simulink model "Assignment_lego"  (R2023b)
settings: Solver=FixedStepAuto  StartTime=0.0  StopTime=10  RelTol=1e-3  EnableMultiTasking=on
libraries: legoev3lib x7
settings Model: ExtModeBatchMode=on  ExtModeTrigDuration=2  Creator=Krish  LastModifiedBy=Krish
settings SolverCC: PositivePriorityOrder=on  AutoInsertRateTranBlk=on
settings OptimizationCC: EnhancedBackFolding=on  PassReuseOutputArgsAs=Individual arguments  ZeroExternalMemoryAtStartup=off  ZeroInternalMemoryAtStartup=off  MaxStackSize=64  OptimizeBlockOrder=speed  DifferentSizesBufferReuse=on  OptimizationCustomize=off  EfficientTunableParamExpr=on
settings DebuggingCC: ParameterTunabilityLossMsg=error
settings HardwareCC: ProdBitPerPointer=32  ProdBitPerSizeT=32  ProdBitPerPtrDiffT=32  ProdLargestAtomicInteger=Long  ProdWordSize=32  ProdHWDeviceType=ARM Compatible->ARM 9
settings SFSimCC: MATLABDynamicMemAlloc=off
settings RTWCC: Description=Embedded Coder  SystemTargetFile=ert.tlc  HardwareBoard=LEGO MINDSTORMS EV3  TLCOptions="-aInlineSetEventsForThisBaseRateFcn=TLC_FALSE -aSuppressMultiTaskScheduler=TLC_FALSE  -aRateBasedStepFcn=0"  TemplateMakefile=ert_default_tmf  Toolchain=Sourcery G++ Lite v2009q3
settings CodeAppCC: ForceParamTrailComments=on  IgnoreCustomStorageClasses=off  OperatorAnnotations=on  SimulinkDataObjDesc=on  SFDataObjDesc=on  InsertBlockDesc=on
settings ERTTargetCC: SupportContinuousTime=on  SupportVariableSizeSignals=on  ExtModeTransport=2  ExtModeStaticAlloc=on  ExtModeMexFile=ext_xcp  ExtModeIntrfLevel=Level2 - Open

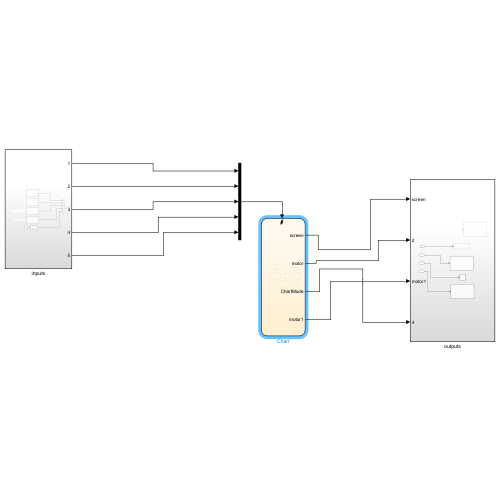
[thumbnail: Simulink's stored preview of the top-level diagram]
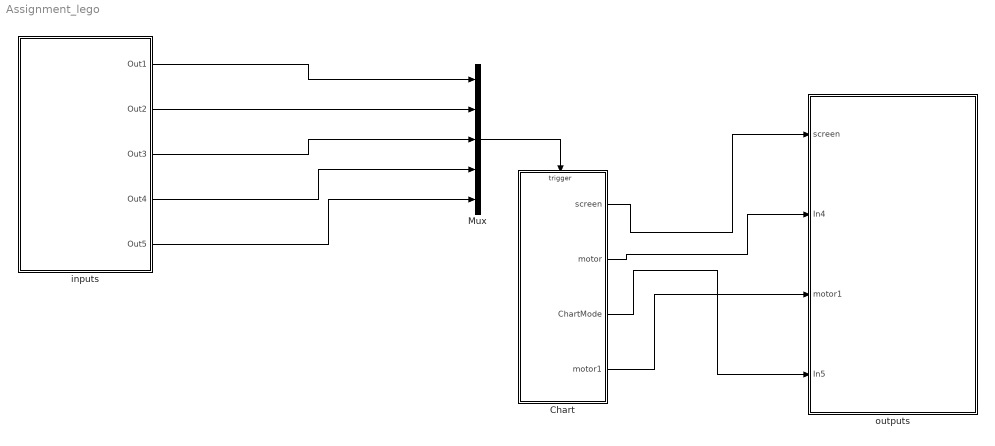
== system Assignment_lego ==
  Chart : Stateflow chart  TreatAsAtomicUnit=on
  Mux : Mux  Inputs=5
  inputs : Subsystem
  outputs : Subsystem
  wires:
  Mux/1 -> Chart/Trigger
  inputs/1(Out1) -> Mux/1
  inputs/2(Out2) -> Mux/2
  inputs/3(Out3) -> Mux/3
  inputs/4(Out4) -> Mux/4
  inputs/5(Out5) -> Mux/5
  Chart/1(screen) -> outputs/1(screen)
  Chart/2(motor) -> outputs/2(In4)
  Chart/3(ChartMode) -> outputs/4(In5)
  Chart/4(motor1) -> outputs/3(motor1)

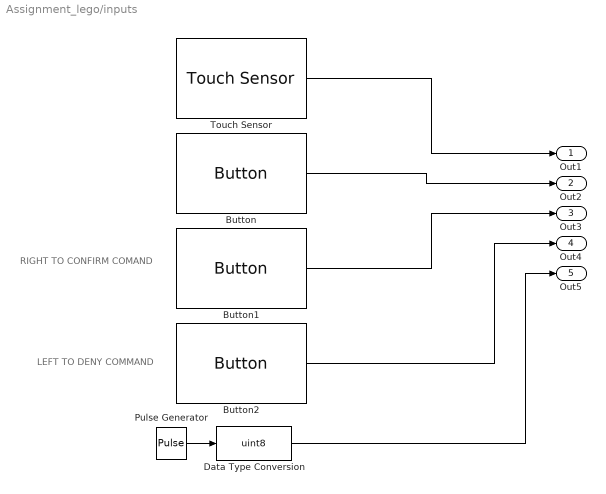
== system Assignment_lego/inputs ==
  note: LEFT TO DENY COMMAND
  note: RIGHT TO CONFIRM COMAND
  Button : legoev3lib/Button  buttonType=Center  sampleTime=0.1
  Button1 : legoev3lib/Button  buttonType=Right  sampleTime=0.1
  Button2 : legoev3lib/Button  buttonType=Left  sampleTime=0.1
  Data Type Conversion : DataTypeConversion  OutDataTypeStr=uint8  SaturateOnIntegerOverflow=off  RndMeth=Floor
  Pulse Generator : DiscretePulseGenerator  Period=10  PulseWidth=2
  Touch Sensor : legoev3lib/Touch Sensor  portNumber=1  sampleTime=0.1
  Out1 : Outport
  Out2 : Outport  Port=2
  Out3 : Outport  Port=3
  Out4 : Outport  Port=4
  Out5 : Outport  Port=5
  wires:
  Pulse Generator/1 -> Data Type Conversion/1
  Button/1 -> Out2/1
  Button2/1 -> Out4/1
  Button1/1 -> Out3/1
  Data Type Conversion/1 -> Out5/1
  Touch Sensor/1 -> Out1/1

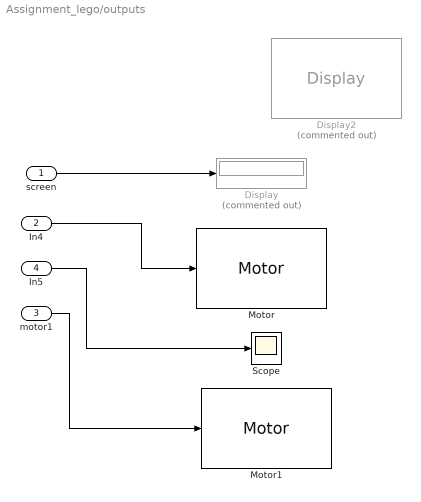
== system Assignment_lego/outputs ==
  screen : Inport
  In4 : Inport  Port=2
  motor1 : Inport  Port=3
  In5 : Inport  Port=4
  Display : Display  Commented=on
      settings: Format=long_e
  Display2 : legoev3lib/Display  Commented=on  slcdStr=Idle  slcdLine=1  slcdFormat=Decimal
  Motor : legoev3lib/Motor  sportNumber=A  sstopAction=Brake
  Motor1 : legoev3lib/Motor  sportNumber=B  sstopAction=Brake
  Scope : Scope
  wires:
  In4/1 -> Motor/1
  In5/1 -> Scope/1
  screen/1 -> Display/1
  motor1/1 -> Motor1/1

== stateflow chart Assignment_lego/Chart ==
  settings: executeAtInitialization=1
  state Confirmation1
    entry:
    screen = "confirm";
  state Off
    entry:
    motor=0;
    during:
    screen="Stopped";
  state OFF2
    during:
    motor=0;
    motor1=0;
  state On1
    entry:
    motor =100;
    motor1=100;
    during:
    screen="Running";
  state Confirmation
    entry:
    screen = "confirm?";
  state EmergencyStop
    entry:
    motor=0;
    during:
    screen="Emergency_stop";
  state mid_state
  Confirmation1 -> (junction 50) [order 2] : confirm{screen="confrimed"}
  (junction 50) -> Off
  Confirmation1 -> On1 [order 1] : deny{screen="denided"}
  On1 -> Confirmation1 [order 2] : Center_btn_pressed
  (default) -> Off
  Confirmation -> Off [order 3] : confirm{screen="confrimed"}
  On1 -> OFF2 [order 4] : after(2.1,sec)
  On1 -> Confirmation [order 3] : Center_btn_pressed
  Confirmation -> Off [order 2] : deny{screen="denied"}
  Off -> Confirmation : Center_btn_pressed
  Confirmation -> On1 [order 1] : confirm{screen="confrimed"}
  (junction 101) -> On1
  On1 -> (junction 83) [order 1]
  (junction 83) -> EmergencyStop : e_btnPressed{screen="Emergency Stop"}
  EmergencyStop -> (junction 90)
  (junction 91) -> EmergencyStop
  (junction 90) -> mid_state : e_btnPressed
  mid_state -> (junction 101) [order 2] : e_btnPressed
  mid_state -> (junction 91) [order 1] : after(4,sec)
  data: screen output string =0; motor output =0; ChartMode output Enum: ChartModeType; motor1 output
  events: e_btnPressed input RISING_EDGE_EVENT; Center_btn_pressed input RISING_EDGE_EVENT; confirm input RISING_EDGE_EVENT; deny input RISING_EDGE_EVENT; clock input RISING_EDGE_EVENT
